simulink model "sltbu"  (R2018a)
settings: Solver=ode3  StartTime=0.0  StopTime=999999  FixedStep=0.1  MaxStep=0.1  RelTol=1e-3  AbsTol=1e-6
PreLoadFcn:
  | inittbu;
model workspace (MAT data in the model file):
  Speed = Simulink.Signal
  Speed.DataType = 'double'
  Speed.Dimensions = -1
  Speed.DimensionsMode = 'auto'
  Speed.Complexity = 'real'
  Speed.SampleTime = -1
  Speed.SamplingMode = 'auto'
  Speed.InitialValue = '1'
undefined symbols (not defined in the file): backup_speed, TbuInitCond, truck_l
libraries: fuzblock x1
CloseFcn:
  | [winName] = get_param(0, 'CurrentSystem'); AnimFigTitle = [winName, ': Truck Backer-Upper Animation']; AnimFigH = findobj(0,'Name',AnimFigTitle); close(AnimFigH)
settings Model: FPTRunName=Active  Creator=The MathWorks, Inc.  LastModifiedBy=22711
settings SolverCC: AutoScaleAbsTol=off
settings DataIOCC: SaveFormat=Array  SaveOutput=off  SaveTime=off
settings OptimizationCC: BlockReduction=off  BooleanDataType=off  ExpressionDepthLimit=2147483647  InitFltsAndDblsToZero=on  LifeSpan=inf
settings DebuggingCC: SaveWithParameterizedLinksMsg=none  UnderspecifiedInitializationDetection=Classic  MergeDetectMultiDrivingBlocksExec=none  SignalResolutionControl=TryResolveAllWithWarning  MultiTaskDSMMsg=warning  MultiTaskCondExecSysMsg=none  FcnCallInpInsideContextMsg=warning  StateNameClashWarn=warning  SFUnexpectedBacktrackingDiag=warning  SFNoUnconditionalDefaultTransitionDiag=warning  SFExecutionAtInitializationDiag=none
settings HardwareCC: ProdBitPerPointer=32  ProdBitPerSizeT=32  ProdBitPerPtrDiffT=32  ProdLargestAtomicFloat=None  ProdIntDivRoundTo=Undefined  ProdEndianess=Unspecified  ProdWordSize=32  ProdHWDeviceType=32-bit Generic  TargetUnknown=on
settings ModelReferenceCC: PropagateSignalLabelsOutOfModel=off
settings RTWCC: TemplateMakefile=grt_vc.tmf
settings CodeAppCC: StateflowObjectComments=on
settings GRTTargetCC: TargetFcnLib=ansi_tfl_tmw.mat  TargetLangStandard=C89/C90 (ANSI)  GeneratePreprocessorConditionals=Disable all  CombineOutputUpdateFcns=off  GRTInterface=on
settings ConfigComp: CovMetricSettings=dw  CovHtmlReporting=on  CovSaveCumulativeToWorkspaceVar=on  CovSaveSingleToWorkspaceVar=on  CovExternalEMLEnable=off

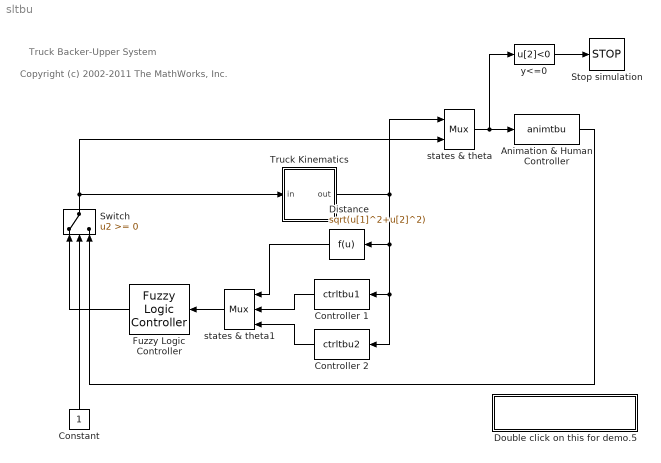
== system sltbu ==
  note: Copyright (c) 2002-2011 The MathWorks, Inc.
  note: Truck Backer-Upper System
  " Animation & Human Controller" : S-Function  FunctionName=animtbu  SFunctionDeploymentMode=off  EnableBusSupport=off
  Constant : Constant
  Controller 1 : MATLABFcn  MATLABFcn=ctrltbu1  OutputDimensions=1
  Controller 2 : MATLABFcn  MATLABFcn=ctrltbu2  OutputDimensions=1
  Distance : Fcn  Expr=sqrt(u[1]^2+u[2]^2)
  Double click on this for demo.5 : Subsystem
      settings: OpenFcn=inittbu
      mask Display: disp('Variable Initialization')
  Fuzzy Logic Controller : fuzblock/Fuzzy Logic  Controller  FIS=fismat  OutputSampleNumber=101  DataType=double  FuzzifiedInputs=off  RuleFiringStrengths=off  RuleOutputs=off  AggregatedOutputs=off  SimulateUsing=Interpreted execution  OutOfRangeInputValueMessage=warning  NoRuleFiredMessage=warning  EmptyOutputFuzzySetMessage=warning
  Stop simulation : Stop
  Switch : Switch  SaturateOnIntegerOverflow=on  InputSameDT=on
  Truck Kinematics : Subsystem  mask(Truck Dynamics){init_cond=TbuInitCond, backup_speed=backup_speed, truck_l=truck_l}
      mask prompts: init_cond "Initial Conditions (x, y, phi):"; backup_speed "Backup Speed:"; truck_l "truck Length:"
      mask help: Truck Dynamics
      mask Help: Truck dynamics
      mask Display: plot(-3, -3, 3, 3,[-1 1 1 -1 -1],[-2 -2 2 2 -2],[-1.1 -1.1],[-2 -1],[1.1 1.1],[-2 -1],[1.35 0.85],[1.93 1.07],[-0.85 -1.35],[1.93 1.07])
  states & theta : Mux  Inputs=[3 1]
  states & theta1 : Mux  Inputs=3
  y<=0 : Fcn  Expr=u[2]<0
  wires:
  y<=0/1 -> Stop simulation/1
  Switch/1 -> states & theta/2, Truck Kinematics/1(in)
  Truck Kinematics/1(out) -> states & theta/1, Distance/1, Controller 1/1, Controller 2/1
  Constant/1 -> Switch/2
  states & theta/1 -> " Animation & Human Controller"/1, y<=0/1
  Fuzzy Logic Controller/1 -> Switch/1
  " Animation & Human Controller"/1 -> Switch/3
  states & theta1/1 -> Fuzzy Logic Controller/1
  Controller 1/1 -> states & theta1/2
  Controller 2/1 -> states & theta1/3
  Distance/1 -> states & theta1/1

== system sltbu/Double click on this for demo.5 ==

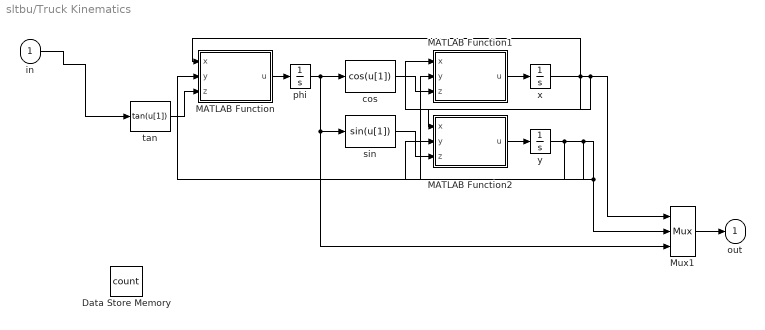
== system sltbu/Truck Kinematics ==
  in : Inport
  Data Store Memory : DataStoreMemory  DataStoreName=count  ReadBeforeWriteMsg=warning  WriteAfterWriteMsg=warning  WriteAfterReadMsg=warning  ShowAdditionalParam=off  OutDataTypeStr=double
  MATLAB Function : MATLAB Function  TreatAsAtomicUnit=on
  MATLAB Function1 : MATLAB Function  TreatAsAtomicUnit=on
  MATLAB Function2 : MATLAB Function  TreatAsAtomicUnit=on
  Mux1 : Mux  Inputs=3
  cos : Fcn  Expr=cos(u[1])
  phi : Integrator  InitialCondition=init_cond(3)
  sin : Fcn
  tan : Fcn  Expr=tan(u[1])
  x : Integrator  InitialCondition=init_cond(1)
  y : Integrator  InitialCondition=init_cond(2)
  out : Outport  InitialOutput=0
  wires:
  phi/1 -> sin/1, Mux1/3, cos/1
  MATLAB Function2/1(u) -> y/1
  Mux1/1 -> out/1
  x/1 -> MATLAB Function/1(x), MATLAB Function1/1(x), MATLAB Function2/1(x), Mux1/1
  y/1 -> MATLAB Function/2(y), MATLAB Function1/2(y), MATLAB Function2/2(y), Mux1/2
  in/1 -> tan/1
  MATLAB Function/1(u) -> phi/1
  MATLAB Function1/1(u) -> x/1
  sin/1 -> MATLAB Function2/3(z)
  tan/1 -> MATLAB Function/3(z)
  cos/1 -> MATLAB Function1/3(z)

== matlab function sltbu/Truck Kinematics/MATLAB Function1 ==
  settings: updateMethod=DISCRETE
  data: x input; y input; u output; z input; count data_store_memory
function u=fcn(x,y,z)
%#codegen
global count;
dis=sqrt(x*x+y*y);
speed=dis;
if count==1
 if dis > 50
     speed = sqrt(x*x+y*y);
 else
     if dis>25
     speed = exp(sqrt(x*x+y*y)/50);
     else
         speed = exp(sqrt(x*x+y*y)/100);
     end
 end
 u=z*(-speed/8);
else
    u=z*0.1;
end

== matlab function sltbu/Truck Kinematics/MATLAB Function ==
  settings: updateMethod=DISCRETE
  data: x input; y input; u output; z input; count data_store_memory
function u=fcn(x,y,z)
%#codegen
global count;
dis=sqrt(x*x+y*y);
speed=dis;
if y>4
    count=1;
end
if count==1
 if dis > 50
     speed = sqrt(x*x+y*y);
 else
     if dis>25
     speed = exp(sqrt(x*x+y*y)/50);
     else
         speed = exp(sqrt(x*x+y*y)/100);
     end
 end
 u=z*(-speed/8);
else
    u=z*0.1/4;
end

== matlab function sltbu/Truck Kinematics/MATLAB Function2 ==
  settings: updateMethod=DISCRETE
  data: x input; y input; u output; z input; count data_store_memory
function u=fcn(x,y,z)
%#codegen
global count;
dis=sqrt(x*x+y*y);
speed=dis;
if count==1
 if dis > 50
     speed = sqrt(x*x+y*y);
 else
     if dis>25
     speed = exp(sqrt(x*x+y*y)/50);
     else
         speed = exp(sqrt(x*x+y*y)/100);
     end
 end
 u=z*(-speed/8);
else
    u=z*0.1;
end
